simulink model "udp_send"  (R2013a)
settings: Solver=ode3  StartTime=0.0  StopTime=inf  FixedStep=DT  RelTol=1e-3
InitFcn:
  | DT = 0.01;
libraries: etargetslib x2, dspnetwork x1
settings Model: Creator=Nima  LastModifiedBy=Nima

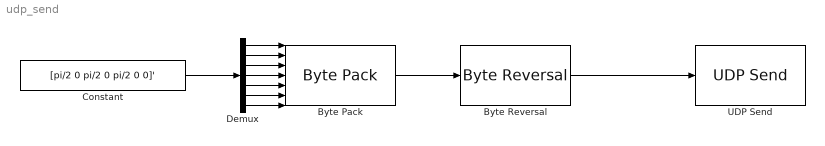
== system udp_send ==
  Byte Pack : etargetslib/Byte Pack  datatypes={'double' 'double' 'double' 'double' 'double' 'double' 'double'}  byteAlign=1
  Byte Reversal : etargetslib/Byte Reversal  numInp=1
  Constant : Constant  Value=[pi/2 0 pi/2 0 pi/2 0 0]'  VectorParams1D=off  SampleTime=DT
  Demux : Demux  Outputs=7
  UDP Send : dspnetwork/UDP Send  remoteURL='127.0.0.1'  remotePort=32000  localURL='255.255.255.255'  localPortSource=Automatically determine  localPort=-1  sampletime=-1  blockPlatform=HOST  separateLengthPort=0
  wires:
  Byte Pack/1 -> Byte Reversal/1
  Demux/1 -> Byte Pack/1
  Demux/2 -> Byte Pack/2
  Demux/5 -> Byte Pack/5
  Demux/7 -> Byte Pack/7
  Demux/6 -> Byte Pack/6
  Demux/4 -> Byte Pack/4
  Demux/3 -> Byte Pack/3
  Constant/1 -> Demux/1
  Byte Reversal/1 -> UDP Send/1
